simulink model "simulinkForce"  (R2017a)
settings: Solver=ode15s  StartTime=0.0  StopTime=5  RelTol=1e-3
PreLoadFcn:
  | % Friction force law lookup table data
  | frictForce = [-35 -25 -30 30 25 35];
  | frictSpeed = [-1 -0.02 -0.01 0.01 0.02 1];
settings Model: Creator=scastro  LastModifiedBy=scastro
settings DebuggingCC: UnderspecifiedInitializationDetection=Classic  MergeDetectMultiDrivingBlocksExec=none
settings ModelReferenceCC: PropagateSignalLabelsOutOfModel=off

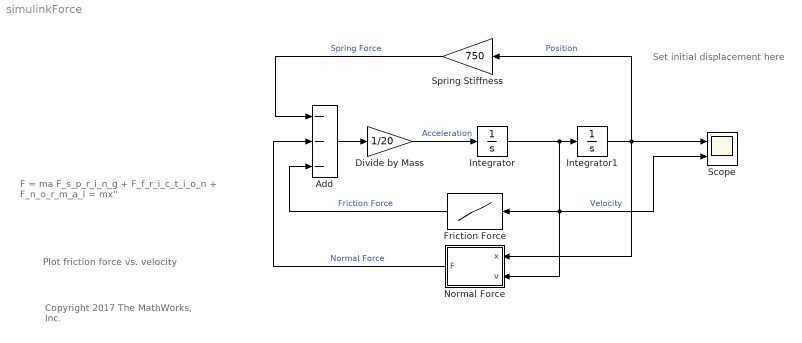
== system simulinkForce ==
  note: Copyright 2017 The MathWorks, Inc.
  note: Plot friction force vs. velocity
  note: Set initial displacement here
  note: F = ma
      |
      | F_s_p_r_i_n_g + F_f_r_i_c_t_i_o_n + F_n_o_r_m_a_l = mx''
  Add : Sum  Inputs=---
  Divide by Mass : Gain  Gain=1/20
  Friction Force : Lookup_n-D  NumberOfTableDimensions=1  BreakpointsForDimension1=frictSpeed  Table=frictForce  InternalRulePriority=Speed  RndMeth=Simplest  InputSameDT=on
  Integrator : Integrator
  Integrator1 : Integrator  InitialCondition=1
  Normal Force : Subsystem
  Scope : Scope  NumInputPorts=2
  Spring Stiffness : Gain  Gain=750
  wires:
  Integrator/1 -> Friction Force/1, Scope/2, Normal Force/2(v), Integrator1/1  "Velocity"
  Integrator1/1 -> Normal Force/1(x), Scope/1, Spring Stiffness/1  "Position"
  Spring Stiffness/1 -> Add/1  "Spring Force"
  Add/1 -> Divide by Mass/1
  Normal Force/1(F) -> Add/2  "Normal Force"
  Divide by Mass/1 -> Integrator/1  "Acceleration"
  Friction Force/1 -> Add/3  "Friction Force"

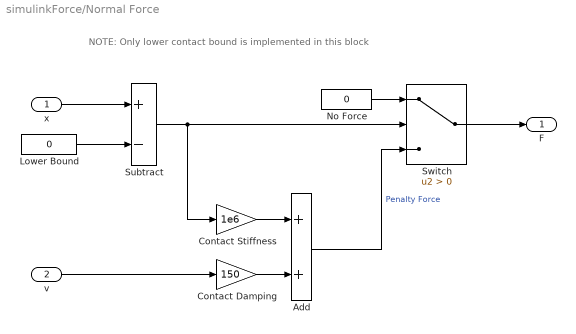
== system simulinkForce/Normal Force ==
  note: NOTE: Only lower contact bound is implemented in this block
  x : Inport
  v : Inport  Port=2
  Add : Sum
  Contact Damping : Gain  Gain=150
  Contact Stiffness : Gain  Gain=1e6
  Lower Bound : Constant  Value=0
  No Force : Constant  Value=0
  Subtract : Sum  Inputs=+-
  Switch : Switch  Criteria=u2 > Threshold
  F : Outport
  wires:
  x/1 -> Subtract/1
  Subtract/1 -> Contact Stiffness/1, Switch/2
  No Force/1 -> Switch/1
  Lower Bound/1 -> Subtract/2
  Contact Stiffness/1 -> Add/1
  Add/1 -> Switch/3  "Penalty Force"
  v/1 -> Contact Damping/1
  Contact Damping/1 -> Add/2
  Switch/1 -> F/1
